simulink model "sistema"  (R2023a)
settings: Solver=ode15s  StartTime=0.0  StopTime=40  RelTol=1e-3
settings Model: Creator=sm13m  LastModifiedBy=sm13m
settings DataIOCC: SaveOutput=off  SignalLogging=off  DSMLogging=off  ReturnWorkspaceOutputs=off  TimeSaveName=t
settings DebuggingCC: AlgebraicLoopMsg=none  ArtificialAlgebraicLoopMsg=none  MaxConsecutiveZCsMsg=none  ModelReferenceExtraNoncontSigs=none  OperatingPointInterfaceChecksumMismatchMsg=none

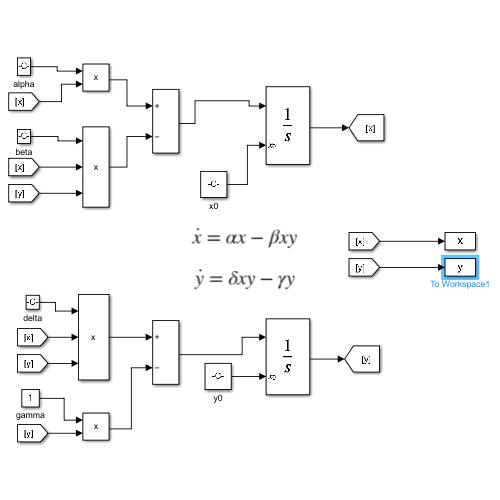
[thumbnail: Simulink's stored preview of the top-level diagram]
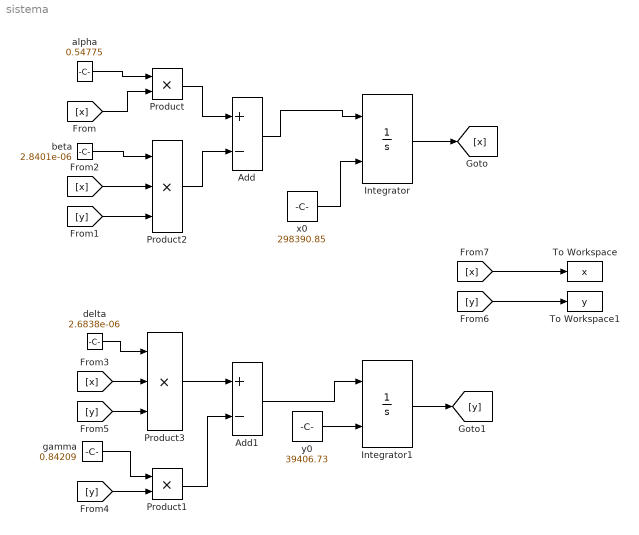
== system sistema ==
  Add : Sum  Inputs=+-
  Add1 : Sum  Inputs=+-
  Integrator : Integrator  InitialConditionSource=external
  Integrator1 : Integrator  InitialConditionSource=external
  Product : Product
  Product1 : Product
  Product2 : Product  Inputs=3
  Product3 : Product  Inputs=3
  To Workspace : ToWorkspace  VariableName=x  SampleTime=-1
  To Workspace1 : ToWorkspace  VariableName=y  SampleTime=-1
  alpha : Constant  Value=0.54775
  beta : Constant  Value=2.8401e-06
  delta : Constant  Value=2.6838e-06
  gamma : Constant  Value=0.84209
  x0 : Constant  Value=298390.85
  y0 : Constant  Value=39406.73
  wires:
  Add/1 -> Integrator/1
  Add1/1 -> Integrator1/1
  x0/1 -> Integrator/2
  y0/1 -> Integrator1/2
  Product/1 -> Add/1
  Product2/1 -> Add/2
  Product1/1 -> Add1/2
  Product3/1 -> Add1/1
  [y] -> Product2/3
  [x] -> Product2/2
  beta/1 -> Product2/1
  alpha/1 -> Product/1
  [x] -> Product/2
  gamma/1 -> Product1/1
  [y] -> Product1/2
  delta/1 -> Product3/1
  [x] -> Product3/2
  [y] -> Product3/3
  Integrator/1 -> [x]
  Integrator1/1 -> [y]
  [x] -> To Workspace/1
  [y] -> To Workspace1/1
